simulink library "openLoopPathDomainCtrl_cl"  (R2018b)
settings: Solver=VariableStepAuto  StartTime=0.0  StopTime=10.0  RelTol=1e-3
undefined symbols (not defined in the file): initialPathPosition_none
libraries: pathProjection_ul x1
settings Model: Creator=mcobb  LastModifiedBy=mitch
settings DebuggingCC: LibraryContextMissingDiagnostic=none
settings SFSimCC: SimUseLocalCustomCode=off
settings RTWCC: RTWUseLocalCustomCode=off

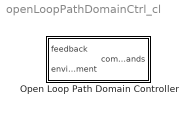
== system openLoopPathDomainCtrl_cl ==
  Open Loop Path Domain Controller : Subsystem  VariantControl=VSS_OPENLOOP_CTRL

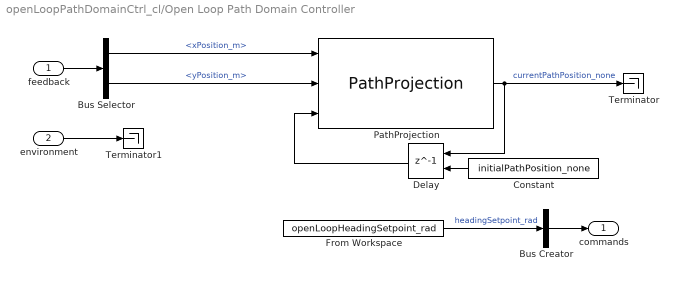
== system openLoopPathDomainCtrl_cl/Open Loop Path Domain Controller ==
  feedback : Inport
  environment : Inport  Port=2
  Bus Creator : BusCreator  Inputs=1
  Bus Selector : BusSelector  OutputSignals=xPosition_m,yPosition_m
  Constant : Constant  Value=initialPathPosition_none
  Delay : Delay  DelayLength=1  InitialConditionSource=Input port
      settings: InputPortMap=u0,p4
  From Workspace : FromWorkspace  VariableName=openLoopHeadingSetpoint_rad  SampleTime=0
  PathProjection : pathProjection_ul/PathProjection  SystemSampleTime=-1
  Terminator : Terminator
  Terminator1 : Terminator
  commands : Outport
  wires:
  environment/1 -> Terminator1/1
  From Workspace/1 -> Bus Creator/1  "headingSetpoint_rad"
  Bus Creator/1 -> commands/1
  feedback/1 -> Bus Selector/1
  Bus Selector/1 -> PathProjection/1  "<xPosition_m>"
  Bus Selector/2 -> PathProjection/2  "<yPosition_m>"
  PathProjection/1 -> Delay/1, Terminator/1  "currentPathPosition_none"
  Delay/1 -> PathProjection/3
  Constant/1 -> Delay/2
